simulink model "LQRAirrefueling"  (R2013a)
settings: Solver=ode45  StartTime=0.0  StopTime=50  RelTol=1e-3
values from neighbouring files (symbols this model uses):
  A1 = [0	0 393.72	0	-393.72	0	0	0 ... (first row only)    [LQR_Calc2.m]    (also in LQR_Calc2LowPrecision.m = [0	0	393.72	0	-393.72	0	0	0; LQR_Calc2_F16YingHu.m = [0   1   0   0   0   0   0)
  B1 = [0	0 ... (first row only)    [LQR_Calc2.m]    (also in LQR_Calc2LowPrecision.m; LQR_Calc2_F16YingHu.m = [ 0  0)
  C_v_theta = C1(1:2,:)    [LQR_Calc2.m]    (also in LQR_Calc2LowPrecision.m)
  Ki = zeros(4,3)    [F16NolinearModelRemoveWindControlData_low.m]    (also in F16_2003hiModelAutopilot.m; F16_2003hiModelAutopilot1.m; LQR_Calc2.m = -k(:,9:10); LQR_Calc2LowPrecision.m = -k(:,9:10))
  Kp = zeros(4,18)    [F16NolinearModelRemoveWindControlData_low.m]    (also in F16_2003hiModelAutopilot.m; F16_2003hiModelAutopilot1.m; F16_2003hiModelAutopilot1_steadySys.m; LQR_Calc2.m = k(:,1:8))
libraries: simulink x2
settings Model: Creator=Dai  LastModifiedBy=Dai

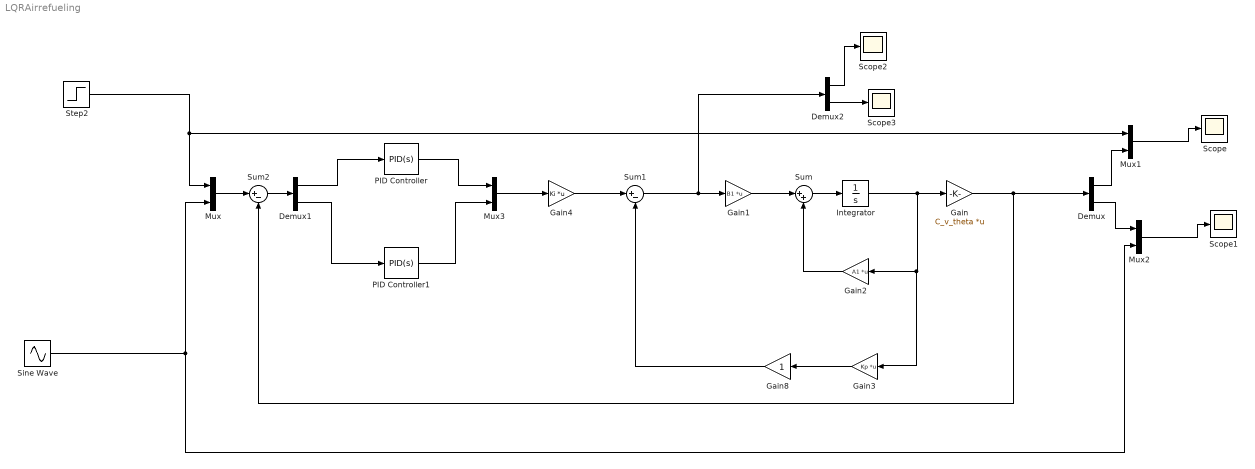
== system LQRAirrefueling ==
  Demux : Demux  Outputs=2
  Demux1 : Demux  Outputs=2
  Demux2 : Demux  Outputs=2
  Gain : Gain  Gain=C_v_theta  Multiplication=Matrix(K*u) (u vector)
  Gain1 : Gain  Gain=B1  Multiplication=Matrix(K*u) (u vector)
  Gain2 : Gain  Gain=A1  Multiplication=Matrix(K*u) (u vector)
  Gain3 : Gain  Gain=Kp  Multiplication=Matrix(K*u) (u vector)
  Gain4 : Gain  Gain=Ki  Multiplication=Matrix(K*u) (u vector)
  Gain8 : Gain
  Integrator : Integrator
  Mux{,1..3} (4 alike) : Mux  Inputs=2
  PID Controller : simulink/Continuous/PID Controller  Controller=PID  TimeDomain=Continuous-time  SampleTime=1  IntegratorMethod=Forward Euler  FilterMethod=Forward Euler  Form=Parallel  P=0  I=1  D=0  N=100  InitialConditionSource=internal  InitialConditionForIntegrator=0  InitialConditionForFilter=0  ExternalReset=none  LimitOutput=off  UpperSaturationLimit=inf  LowerSaturationLimit=-inf  LinearizeAsGain=on  AntiWindupMode=none  Kb=1  TrackingMode=off  Kt=1  PParamMin=[]  PParamMax=[]  IParamMin=[]  IParamMax=[]  DParamMin=[]  DParamMax=[]  NParamMin=[]  NParamMax=[]  KbParamMin=[]  KbParamMax=[]  KtParamMin=[]  KtParamMax=[]  POutMin=[]  POutMax=[]  IOutMin=[]  IOutMax=[]  DOutMin=[]  DOutMax=[]  NOutMin=[]  NOutMax=[]  KbOutMin=[]  KbOutMax=[]  KtOutMin=[]  KtOutMax=[]  IntegratorOutMin=[]  IntegratorOutMax=[]  FilterOutMin=[]  FilterOutMax=[]  SumOutMin=[]  SumOutMax=[]  SumI1OutMin=[]  SumI1OutMax=[]  SumI2OutMin=[]  SumI2OutMax=[]  SumI3OutMin=[]  SumI3OutMax=[]  SumDOutMin=[]  SumDOutMax=[]  SaturationOutMin=[]  SaturationOutMax=[]  IntegratorContinuousStateAttributes=''  IntegratorStateMustResolveToSignalObject=off  IntegratorRTWStateStorageClass=Auto  FilterContinuousStateAttributes=''  FilterStateMustResolveToSignalObject=off  FilterRTWStateStorageClass=Auto
  PID Controller1 : simulink/Continuous/PID Controller  Controller=PID  TimeDomain=Continuous-time  SampleTime=1  IntegratorMethod=Forward Euler  FilterMethod=Forward Euler  Form=Parallel  P=0  I=1  D=0  N=100  InitialConditionSource=internal  InitialConditionForIntegrator=0  InitialConditionForFilter=0  ExternalReset=none  LimitOutput=off  UpperSaturationLimit=inf  LowerSaturationLimit=-inf  LinearizeAsGain=on  AntiWindupMode=none  Kb=1  TrackingMode=off  Kt=1  PParamMin=[]  PParamMax=[]  IParamMin=[]  IParamMax=[]  DParamMin=[]  DParamMax=[]  NParamMin=[]  NParamMax=[]  KbParamMin=[]  KbParamMax=[]  KtParamMin=[]  KtParamMax=[]  POutMin=[]  POutMax=[]  IOutMin=[]  IOutMax=[]  DOutMin=[]  DOutMax=[]  NOutMin=[]  NOutMax=[]  KbOutMin=[]  KbOutMax=[]  KtOutMin=[]  KtOutMax=[]  IntegratorOutMin=[]  IntegratorOutMax=[]  FilterOutMin=[]  FilterOutMax=[]  SumOutMin=[]  SumOutMax=[]  SumI1OutMin=[]  SumI1OutMax=[]  SumI2OutMin=[]  SumI2OutMax=[]  SumI3OutMin=[]  SumI3OutMax=[]  SumDOutMin=[]  SumDOutMax=[]  SaturationOutMin=[]  SaturationOutMax=[]  IntegratorContinuousStateAttributes=''  IntegratorStateMustResolveToSignalObject=off  IntegratorRTWStateStorageClass=Auto  FilterContinuousStateAttributes=''  FilterStateMustResolveToSignalObject=off  FilterRTWStateStorageClass=Auto
  Scope{,1..3} (4 alike) : Scope
      Scope2 settings: SaveName=ScopeData2
      Scope3 settings: SaveName=ScopeData3
  Sine Wave : Sin  Frequency=0.02  SampleTime=0
  Step2 : Step  Time=0  SampleTime=0
  Sum : Sum  Inputs=|++
  Sum1 : Sum  Inputs=|+-
  Sum2 : Sum  Inputs=|+-
  wires:
  Integrator/1 -> Gain3/1, Gain2/1, Gain/1
  Gain1/1 -> Sum/1
  Sum/1 -> Integrator/1
  Gain2/1 -> Sum/2
  Gain3/1 -> Gain8/1
  Sum1/1 -> Demux2/1, Gain1/1
  Gain4/1 -> Sum1/1
  Gain/1 -> Demux/1, Sum2/2
  Mux/1 -> Sum2/1
  Step2/1 -> Mux/1, Mux1/1
  Demux/1 -> Mux1/2
  Mux1/1 -> Scope/1
  Sine Wave/1 -> Mux/2, Mux2/2
  Mux2/1 -> Scope1/1
  Demux/2 -> Mux2/1
  Gain8/1 -> Sum1/2
  Sum2/1 -> Demux1/1
  Mux3/1 -> Gain4/1
  Demux1/1 -> PID Controller/1
  PID Controller/1 -> Mux3/1
  Demux1/2 -> PID Controller1/1
  PID Controller1/1 -> Mux3/2
  Demux2/1 -> Scope2/1
  Demux2/2 -> Scope3/1
